simulink model "pd_CEA_comparison_test"  (R2018b)
settings: Solver=VariableStepAuto  StartTime=0.0  StopTime=50  RelTol=1e-3
values from neighbouring files (symbols this model uses):
  qd = qd/norm(qd)    [pd_vs_CEA_unittest_init.m]
libraries: control_command_generation_lib x2, satelliteDynamics_lib x2, PD_Controller_Lib x1, SlewAndControlConstrained_Controller_lib x1
settings Model: Creator=colem  LastModifiedBy=colem

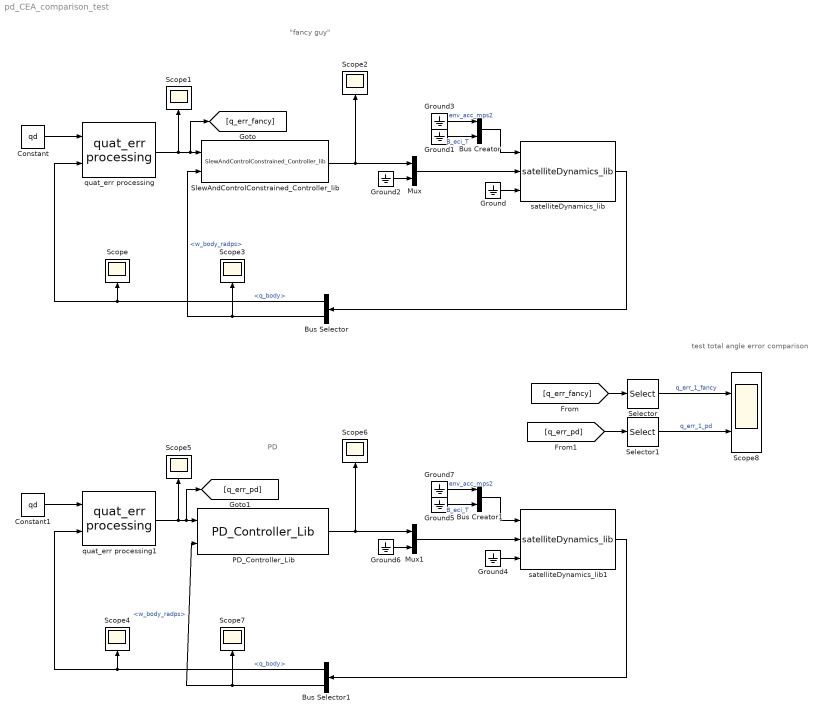
== system pd_CEA_comparison_test ==
  note: test total angle error comparison
  note: PD
  note: "fancy guy"
  Bus Creator : BusCreator  Inputs=2
  Bus Creator1 : BusCreator  Inputs=2
  Bus Selector : BusSelector  OutputSignals=q_body,w_body_radps
  Bus Selector1 : BusSelector  OutputSignals=q_body,w_body_radps
  Constant : Constant  Value=qd
  Constant1 : Constant  Value=qd
  Ground{,1..7} (8 alike) : Ground
  Mux : Mux  Inputs=[3 3]
  Mux1 : Mux  Inputs=[3 3]
  PD_Controller_Lib : PD_Controller_Lib/PD_Controller_Lib  SystemSampleTime=-1
  Scope{,1..7} (8 alike) : Scope
  Scope8 : Scope  NumInputPorts=2
  Selector : Selector  InputPortWidth=4  IndexOptions=Index vector (dialog)  Indices=[1]  OutputSizes=1
  Selector1 : Selector  InputPortWidth=4  IndexOptions=Index vector (dialog)  Indices=[1]  OutputSizes=1
  SlewAndControlConstrained_Controller_lib : SlewAndControlConstrained_Controller_lib/SlewAndControlConstrained_Controller_lib  SystemSampleTime=-1
  quat_err processing : control_command_generation_lib/control_command_generation_lib/quat_err processing  SystemSampleTime=-1
  quat_err processing1 : control_command_generation_lib/control_command_generation_lib/quat_err processing  SystemSampleTime=-1
  satelliteDynamics_lib : satelliteDynamics_lib/satelliteDynamics_lib  SystemSampleTime=-1
  satelliteDynamics_lib1 : satelliteDynamics_lib/satelliteDynamics_lib  SystemSampleTime=-1
  wires:
  Bus Selector/2 -> SlewAndControlConstrained_Controller_lib/2, Scope3/1  "<w_body_radps>"
  satelliteDynamics_lib/1 -> Bus Selector/1
  quat_err processing/1 -> [q_err_fancy], SlewAndControlConstrained_Controller_lib/1, Scope1/1
  SlewAndControlConstrained_Controller_lib/1 -> Mux/1, Scope2/1
  Ground2/1 -> Mux/2
  Mux/1 -> satelliteDynamics_lib/2
  Ground/1 -> satelliteDynamics_lib/3
  Bus Creator/1 -> satelliteDynamics_lib/1
  Constant/1 -> quat_err processing/1
  Ground3/1 -> Bus Creator/1  "env_acc_mps2"
  Bus Selector/1 -> quat_err processing/2, Scope/1  "<q_body>"
  Ground1/1 -> Bus Creator/2  "B_eci_T"
  PD_Controller_Lib/1 -> Mux1/1, Scope6/1
  Ground4/1 -> satelliteDynamics_lib1/3
  satelliteDynamics_lib1/1 -> Bus Selector1/1
  Mux1/1 -> satelliteDynamics_lib1/2
  Bus Selector1/1 -> quat_err processing1/2, Scope4/1  "<q_body>"
  Constant1/1 -> quat_err processing1/1
  quat_err processing1/1 -> [q_err_pd], PD_Controller_Lib/1, Scope5/1
  Ground6/1 -> Mux1/2
  Ground5/1 -> Bus Creator1/2  "B_eci_T"
  Ground7/1 -> Bus Creator1/1  "env_acc_mps2"
  Bus Selector1/2 -> PD_Controller_Lib/2, Scope7/1  "<w_body_radps>"
  Bus Creator1/1 -> satelliteDynamics_lib1/1
  [q_err_fancy] -> Selector/1
  [q_err_pd] -> Selector1/1
  Selector/1 -> Scope8/1  "q_err_1_fancy"
  Selector1/1 -> Scope8/2  "q_err_1_pd"
